simulink model "NLPIDVersion2"  (Simulink 7.3)
settings: Solver=ode5  StartTime=0.0  StopTime=inf  FixedStep=0.1  RelTol=1e-3
undefined symbols (not defined in the file): eta1_0_real, v1_0_real, velocitySatValues1
libraries: dspmtrx3 x16, simulink x14, dspindex x5, marine_gnc x4, simulink_extras x1, dspinverses x1
(part 2 of 4)

== system NLPIDVersion2/Main Subsystems/Control/Nonlinear PID/Auxiliary function g_s ==
  g_s eq : Subsystem
  g_s^q eq : Subsystem
  g_s^s eq : Subsystem
  g_s^t eq : Subsystem
  tag scope: gs=global, gs_q=global, gs_s=global, gs_t=global
  wires:
  [fs_t] -> g_s^t eq/2(f_s^t)
  g_s^t eq/1(g_a^t) -> [gs_t]
  [psiLOS_s_2] -> g_s^s eq/4(psi_los^s^2)
  [fs_s] -> g_s^s eq/3(f_s^s)
  g_s^s eq/1(g_s^s) -> [gs_s]
  g_s^q eq/1(g_s^q) -> [gs_q]
  [psiLOS_qs] -> g_s^q eq/4(psi_los^sq)
  [fs_q] -> g_s^q eq/3(f_s^q)
  g_s eq/1(g_s) -> [gs]
  [psiLOS_s] -> g_s^t eq/1(psi_los^s), g_s^s eq/2(psi_los^s), g_s^q eq/2(psi_los^s), g_s eq/2(psi_los^s)
  [fs] -> g_s^s eq/1(f_s), g_s^q eq/1(f_s), g_s eq/1(f_s)

== system NLPIDVersion2/Main Subsystems/Control/Nonlinear PID/Control law ==
  Sum : Sum  Inputs=+++  OutDataType=fixdt(1, 16)  OutScaling=2^-10
  tau_FF : Subsystem
  tau_FL : Subsystem
  tau_PID : Subsystem
  tag scope: ctrl2tau=global
  wires:
  Sum/1 -> [ctrl2tau]
  tau_PID/1(tau_PID) -> Sum/1
  tau_FL/1(tau_FL) -> Sum/2
  tau_FF/1(tau_FF) -> Sum/3

== system NLPIDVersion2/Main Subsystems/Control/Nonlinear PID/R(psi) ==
  -1 : Gain  Gain=-1  ParameterDataType=fixdt(1, 16)  ParameterScaling=2^0  OutDataType=fixdt(1, 16)  OutScaling=2^0
  Mux : Mux  Inputs=9
  R(psi) : Reshape  OutputDimensionality=Customize  OutputDimensions=[3,3]
  R11 : Trigonometry  Operator=cos
  R12 : Trigonometry
  R{13,23,31..32} (4 alike) : Constant  Value=0
  R21 : Trigonometry
  R22 : Trigonometry  Operator=cos
  R33 : Constant
  R^T : dspmtrx3/Transpose  SystemSampleTime=-1  Hermitian=off  overflowFlag=off
  psi : Selector  InputPortWidth=3  IndexOptions=Index vector (dialog)  Indices=[3]  OutputSizes=1
  tag scope: Rpsi=global, Rpsi_T=global
  wires:
  R(psi)/1 -> [Rpsi], R^T/1
  Mux/1 -> R(psi)/1
  psi/1 -> R11/1, R21/1, R12/1, R22/1
  R11/1 -> Mux/1
  R21/1 -> Mux/2
  R31/1 -> Mux/3
  R12/1 -> -1/1
  R22/1 -> Mux/5
  R32/1 -> Mux/6
  R13/1 -> Mux/7
  R33/1 -> Mux/9
  R23/1 -> Mux/8
  -1/1 -> Mux/4
  [eta] -> psi/1
  R^T/1 -> [Rpsi_T]

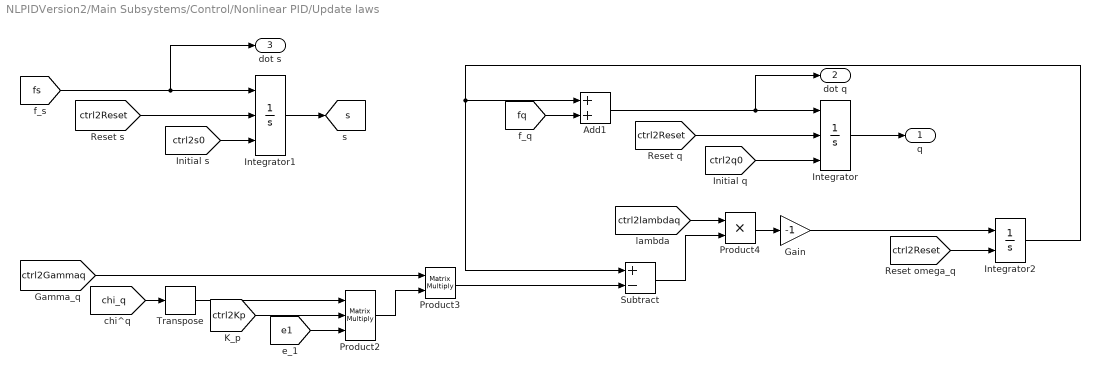
== system NLPIDVersion2/Main Subsystems/Control/Nonlinear PID/Update laws ==
  Add1 : Sum  OutDataType=fixdt(1, 16)  OutScaling=2^-10
  Gain : Gain  Gain=-1  ParameterDataType=fixdt(1, 16)  ParameterScaling=2^0  OutDataType=fixdt(1, 16)  OutScaling=2^0
  Integrator : Integrator  ExternalReset=level  InitialConditionSource=external
  Integrator1 : Integrator  ExternalReset=level  InitialConditionSource=external  InitialCondition=250
  Integrator2 : Integrator  ExternalReset=level
  Product2 : Product  Inputs=3  Multiplication=Matrix(*)  OutDataType=fixdt(1, 16)  OutScaling=2^0  RndMeth=Zero
  Product3 : Product  Multiplication=Matrix(*)  OutDataType=fixdt(1, 16)  OutScaling=2^0  RndMeth=Zero
  Product4 : Product  OutDataType=fixdt(1, 16)  OutScaling=2^0  RndMeth=Zero
  Subtract : Sum  Inputs=+-  OutDataType=fixdt(1, 16)  OutScaling=2^-10
  Transpose : dspmtrx3/Transpose  SystemSampleTime=-1  Hermitian=off  overflowFlag=off
  q : Outport  PortDimensions=2
  dot q : Outport  Port=2  PortDimensions=2
  dot s : Outport  Port=3  PortDimensions=1
  tag scope: s=global
  wires:
  [chi_q] -> Transpose/1
  [e1] -> Product2/3
  Transpose/1 -> Product2/1
  [ctrl2Kp] -> Product2/2
  [ctrl2Gammaq] -> Product3/1
  Product3/1 -> Subtract/2
  Product2/1 -> Product3/2
  [fs] -> Integrator1/1, dot s/1
  Integrator1/1 -> [s]
  [ctrl2Reset] -> Integrator1/2
  [ctrl2s0] -> Integrator1/3
  [fq] -> Add1/2
  Add1/1 -> Integrator/1, dot q/1
  [ctrl2lambdaq] -> Product4/1
  Subtract/1 -> Product4/2
  Product4/1 -> Gain/1
  Gain/1 -> Integrator2/1
  Integrator/1 -> q/1
  Integrator2/1 -> Add1/1, Subtract/1
  [ctrl2Reset] -> Integrator/2
  [ctrl2q0] -> Integrator/3
  [ctrl2Reset] -> Integrator2/2

== system NLPIDVersion2/Main Subsystems/Control/Nonlinear PID/a_d ==
  dot q : Inport
  dot s : Inport  Port=2
  Product : Product  Multiplication=Matrix(*)  OutDataType=fixdt(1, 16)  OutScaling=2^0  RndMeth=Zero
  Product1 : Product  Multiplication=Matrix(*)  OutDataType=fixdt(1, 16)  OutScaling=2^0  RndMeth=Zero
  Sum : Sum  Inputs=+++  OutDataType=fixdt(1, 16)  OutScaling=2^-10
  v_d^q : Subsystem
  v_d^s : Subsystem
  v_d^t : Subsystem
  tag scope: ad=global
  wires:
  v_d^q/1(v_d^q) -> Product/1
  dot q/1 -> Product/2
  Product/1 -> Sum/1
  v_d^s/1(v_d^s) -> Product1/1
  dot s/1 -> Product1/2
  Product1/1 -> Sum/2
  v_d^t/1(v_d^t) -> Sum/3
  Sum/1 -> [ad]
  [gq_q] -> v_d^q/1(g_q^q)
  [gs_q] -> v_d^q/2(g_s^q)
  [gq_s] -> v_d^s/1(g_q^s)
  [gs_s] -> v_d^s/2(g_s^s)
  [gq_t] -> v_d^t/1(g_q^t)
  [gs_t] -> v_d^t/2(g_s^t)

== system NLPIDVersion2/Main Subsystems/Control/Nonlinear PID/e2 ==
  Product : Product  Multiplication=Matrix(*)  OutDataType=fixdt(1, 16)  OutScaling=2^0  RndMeth=Zero
  Subtract : Sum  Inputs=+-  OutDataType=fixdt(1, 16)  OutScaling=2^-10
  tag scope: e2=global
  wires:
  [nu] -> Subtract/1
  Product/1 -> Subtract/2
  [Rpsi_T] -> Product/1
  [vd] -> Product/2
  Subtract/1 -> [e2]

== system NLPIDVersion2/Main Subsystems/Control/Nonlinear PID/e_1 ==
  Heading to -pi/pi : Subsystem
  Heading to -pi/pi1 : Subsystem
  Subtract : Sum  Inputs=+-  OutDataType=fixdt(1, 16)  OutScaling=2^-10
  tag scope: e1=global
  wires:
  Subtract/1 -> Heading to -pi/pi1/1(eta rad)
  [eta] -> Heading to -pi/pi/1(eta rad)
  Heading to -pi/pi/1(eta -pi/pi) -> Subtract/1
  Heading to -pi/pi1/1(eta -pi/pi) -> [e1]
  [chi] -> Subtract/2

== system NLPIDVersion2/Main Subsystems/Control/Nonlinear PID/v_d ==
  Add : Sum  OutDataType=fixdt(1, 16)  OutScaling=2^-10
  tag scope: vd=global
  wires:
  [gq] -> Add/1
  [gs] -> Add/2
  Add/1 -> [vd]

== system NLPIDVersion2/Main Subsystems/Control/Nonlinear PID/zeta ==
  Integrator : Integrator  ExternalReset=level  InitialCondition=[0 0 0]'
  Product : Product  Multiplication=Matrix(*)  OutDataType=fixdt(1, 16)  OutScaling=2^0  RndMeth=Zero
  tag scope: zeta=global
  wires:
  [ctrl2Reset] -> Integrator/2
  Product/1 -> Integrator/1
  Integrator/1 -> [zeta]
  [e2] -> Product/2
  [Rpsi] -> Product/1

== system NLPIDVersion2/Main Subsystems/Control/PS3 u input control/Subsystem ==
  u_act : Inport  OutDataType=fixdt(1, 16)  OutScaling=2^0
  Bus Selector : BusSelector  OutputSignals=u_1,u_2,u_3,u_4,u_5
  Mux : Mux  Inputs=5
  f_act to tau : Subsystem
  u_act to f_act : Subsystem
  tau : Outport
  wires:
  u_act/1 -> Bus Selector/1
  f_act to tau/1(tau) -> tau/1
  u_act to f_act/1(f_act) -> f_act to tau/1(f_act)
  Mux/1 -> u_act to f_act/1(u_act)
  Bus Selector/1 -> Mux/1  "<u_1>"
  Bus Selector/2 -> Mux/2  "<u_2>"
  Bus Selector/3 -> Mux/3  "<u_3>"
  Bus Selector/4 -> Mux/4  "<u_4>"
  Bus Selector/5 -> Mux/5  "<u_5>"

== system NLPIDVersion2/Main Subsystems/Control/Thruster allocation/VSP030 BT040 ==
  f_act : Inport
  BT_power_limit : Constant  Value=0.4
  Mux1 : Mux  Inputs=3
  VSP_speeds : Constant  Value=0.3
  f_act to u_act : Subsystem
  TC : Outport  OutDataType=fixdt(1, 16)  OutScaling=2^0
  wires:
  Mux1/1 -> TC/1
  f_act/1 -> f_act to u_act/1(f_act)
  BT_power_limit/1 -> Mux1/2
  VSP_speeds/1 -> Mux1/3
  f_act to u_act/1(u_act) -> Mux1/1

== system NLPIDVersion2/Main Subsystems/Control/Thruster allocation/tau to f_act ==
  tau : Inport
  Product : Product  Multiplication=Matrix(*)  OutDataType=fixdt(1, 16)  OutScaling=2^0  RndMeth=Zero
  Pseudoinverse : dspinverses/Pseudoinverse  wanterr=off
  f_act : Outport
  wires:
  [B] -> Pseudoinverse/1
  Pseudoinverse/1 -> Product/1
  tau/1 -> Product/2
  Product/1 -> f_act/1

== system NLPIDVersion2/Main Subsystems/Guidance/Line-Of-Sight Path-Following/Heading ==
  Demux : Demux  Outputs=2
  Demux1 : Demux  Outputs=2
  Demux2 : Demux  Outputs=2
  psi_d eq : Subsystem
  psi_d^s eq : Subsystem
  psi_d^s^2 eq : Subsystem
  tag scope: psid=global, psid_s=global, psid_s_2=global
  wires:
  psi_d^s eq/3(den) -> psi_d^s^2 eq/2(den)
  psi_d^s eq/2(num) -> psi_d^s^2 eq/1(num)
  Demux2/2 -> psi_d^s^2 eq/8(y_d^s^3)
  Demux2/1 -> psi_d^s^2 eq/7(x_d^s^3)
  psi_d^s^2 eq/1(psi_d^s^2) -> [psid_s_2]
  [pd_s_3] -> Demux2/1
  psi_d^s eq/1(psi_d^s) -> [psid_s]
  Demux1/2 -> psi_d^s^2 eq/6(y_d^s^2), psi_d^s eq/4(y_d^s^2)
  Demux1/1 -> psi_d^s^2 eq/5(x_d^s^2), psi_d^s eq/3(x_d^s^2)
  [pd_s_2] -> Demux1/1
  [pd_s] -> Demux/1
  Demux/2 -> psi_d^s^2 eq/4(y_d^s), psi_d^s eq/2(y_d^s), psi_d eq/2(y_d^s)
  Demux/1 -> psi_d^s^2 eq/3(x_d^s), psi_d^s eq/1(x_d^s), psi_d eq/1(x_d^s)
  psi_d eq/1(psi_d) -> [psid]

== system NLPIDVersion2/Main Subsystems/Guidance/Line-Of-Sight Path-Following/Line-Of-Sight ==
  Dynamic LOS assigment for qdot : Subsystem
  Dynamic assigment for sdot : Subsystem
  Gradient update law for sdot : Subsystem
  LOS heading : Subsystem
  Position error signals : Subsystem
  Subtract : Sum  Inputs=+-  OutDataType=fixdt(1, 16)  OutScaling=2^-10
  Virtual Vessel : Subsystem
  wires:
  Gradient update law for sdot/3(omega_s^s) -> Dynamic assigment for sdot/6(omega_s^s)
  Gradient update law for sdot/2(omega_s^q) -> Dynamic assigment for sdot/5(omega_s^q)
  Position error signals/4(epsilon_n^q) -> Dynamic assigment for sdot/1(epsilon_n^q), LOS heading/4(epsilon_n^q)
  Position error signals/3(epsilon_n^s^2) -> LOS heading/3(epsilon_n^s^2)
  Position error signals/2(epsilon_n^q^2) -> LOS heading/2(epsilon_n^q^2)
  Position error signals/1(epsilon_n^qs) -> LOS heading/1(epsilon_n^qs)
  Position error signals/5(epsilon_n^s) -> Dynamic assigment for sdot/2(epsilon_n^s), LOS heading/5(epsilon_n^s)
  Position error signals/6(epsilon_n) -> LOS heading/6(epsilon_n), Dynamic assigment for sdot/3(epsilon_n)
  Gradient update law for sdot/1(omega_s) -> Dynamic assigment for sdot/4(omega_s)
  Subtract/1 -> Position error signals/1(q - p_d), Gradient update law for sdot/1(q - p_d)
  [q] -> Subtract/1
  [pd] -> Subtract/2

== system NLPIDVersion2/Main Subsystems/Guidance/Line-Of-Sight Path-Following/Path ==
  note: Path Selector == 1: Linear path
      | Path Selector == 0: Ellipse path
  Ellipse path : Subsystem
  Path Switch workaround + limiter : Subsystem
  Straight path : Subsystem

== system NLPIDVersion2/Main Subsystems/Guidance/Line-Of-Sight Path-Following/Speed assigment ==
  Derivative : Derivative
  v_s eq : Subsystem
  v_s^s eq : Subsystem
  v_s^t eq : Subsystem
  tag scope: ud_t=global, vs=global, vs_s=global, vs_t=global
  wires:
  Derivative/1 -> v_s^t eq/2(u_d^t), [ud_t]
  v_s^t eq/1(v_s^t) -> [vs_t]
  [pd_s_2] -> v_s^s eq/4(p_d^s^2)
  [pd_s] -> v_s^s eq/3(p_d^s)
  v_s^s eq/1(v_s^s) -> [vs_s]
  [ud] -> Derivative/1, v_s^s eq/2(u_d), v_s eq/2(u_d)
  [pd_sabs] -> v_s eq/1(|p_d^s|), v_s^s eq/1(|p_d^s|), v_s^t eq/1(|p_d^s|)
  v_s eq/1(v_s) -> [vs]

== system NLPIDVersion2/Main Subsystems/Plant/CSE1 actuator/Bow Thruster ==
  Bow Thruster Direction u_5 : Inport
  Bow Thruster Power : Inport  Port=2
  Add : Sum  Inputs=+++
  BT_D_Gain1 : Gain  Gain=0.02
  BT_D_Gain2 : Gain  Gain=0.02
  BT_L_Gain1 : Gain  Gain=0.02
  BT_L_Gain2 : Gain  Gain=-0.02
  BT_Power_Offset1 : Constant  Value=0.05
  BT_Power_Offset2 : Constant  Value=0.05
  BT_Power_Offset3 : Constant  Value=0.05
  Constant : Constant  Value=0  OutDataType=fixdt(1, 16)  OutScaling=2^0
  Constant1 : Constant  Value=0  OutDataType=fixdt(1, 16)  OutScaling=2^0
  Neg : Gain  Gain=-1  ParameterDataType=fixdt(1, 16)  ParameterScaling=2^0  OutDataType=fixdt(1, 16)  OutScaling=2^0
  SIT PWM0 BT : S-Function  Priority=1  FunctionName=NI_SIT_IO  Parameters=width dtype portnum stime stype btype  EnableBusSupport=off  mask(SIT Outport){portnum=1, width=-1, stime=-1, dtype=auto, stype=auto, btype=0}
      mask prompts: portnum "Port number:"; width "Port dimensions (-1 for dynamically sized):"; stime "Sample time (-1 for inherited):"; dtype "Data type:"; stype "Signal type:"; btype "Block type:"
      mask help: Use this outport on any level of nested subsystems to allow the LabVIEW Simulation Interface Toolkit to map hardware to it.
      mask init:
      | NI_SIT_IO_init;
      settings: CopyFcn=NI_SIT_IO_callbacks(1);  DeleteFcn=NI_SIT_IO_callbacks(2);
      mask StyleString: edit,edit,edit,popup(auto|double|single|int8|uint8|int16|uint16|int32|uint32|boolean),popup(auto|real|complex),edit
      mask CallbackString: NI_SIT_IO_callbacks(3);|||NI_SIT_IO_callbacks(4);||
      mask TabNameString: Parameters,Parameters,Parameters,Parameters,Parameters,Parameters
      mask Display:
      | patch([-x x], [-y y], [.90980 .81960 .32156]);
      | plot([0 -x x 0], [rad -y y rad]);
      | fprintf('SIT%d', portnum);
  Saturation Dynamic : simulink/Discontinuities/Saturation Dynamic  SystemSampleTime=-1  OutMin=[]  OutMax=[]  OutDataTypeStr=Inherit: Same as second input  OutDataType=fixdt(1, 16)  OutScaling=2^-10  DoSatur=off
  Saturation Dynamic1 : simulink/Discontinuities/Saturation Dynamic  SystemSampleTime=-1  OutMin=[]  OutMax=[]  OutDataTypeStr=Inherit: Same as second input  OutDataType=fixdt(1, 16)  OutScaling=2^-10  DoSatur=off
  Saturation Dynamic2 : simulink/Discontinuities/Saturation Dynamic  SystemSampleTime=-1  OutMin=[]  OutMax=[]  OutDataTypeStr=Inherit: Same as second input  OutDataType=fixdt(1, 16)  OutScaling=2^-10  DoSatur=off
  Sum1 : Sum  Inputs=|++
  Sum2 : Sum  Inputs=|++
  Terminator : Terminator
  Terminator1 : Terminator
  wires:
  Bow Thruster Direction u_5/1 -> BT_D_Gain1/1, Saturation Dynamic1/2, BT_D_Gain2/1, Saturation Dynamic2/2
  BT_D_Gain1/1 -> Add/1
  BT_D_Gain2/1 -> Add/3
  BT_Power_Offset1/1 -> Add/2
  Add/1 -> Saturation Dynamic/2
  Bow Thruster Power/1 -> BT_L_Gain2/1, Saturation Dynamic2/1, BT_L_Gain1/1, Neg/1
  Sum1/1 -> Saturation Dynamic/1
  BT_L_Gain1/1 -> Sum1/1
  BT_L_Gain2/1 -> Sum2/1
  Sum2/1 -> Saturation Dynamic/3
  BT_Power_Offset2/1 -> Sum1/2
  BT_Power_Offset3/1 -> Sum2/2
  Saturation Dynamic/1 -> SIT PWM0 BT/1
  Saturation Dynamic2/1 -> Terminator1/1
  Saturation Dynamic1/1 -> Terminator/1
  Constant/1 -> Saturation Dynamic1/1
  Constant1/1 -> Saturation Dynamic2/3
  Neg/1 -> Saturation Dynamic1/3

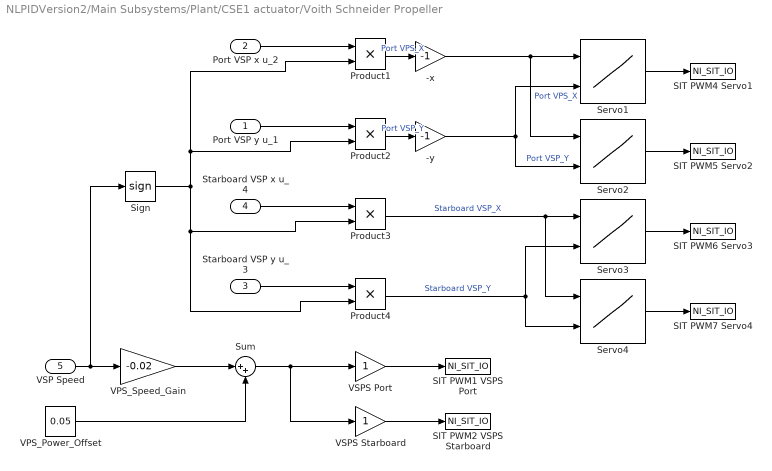
== system NLPIDVersion2/Main Subsystems/Plant/CSE1 actuator/Voith Schneider Propeller  ==
  Port VSP y u_1 : Inport
  Port VSP x u_2 : Inport  Port=2
  Starboard VSP y u_3 : Inport  Port=3
  Starboard VSP x u_4 : Inport  Port=4
  VSP Speed : Inport  Port=5
  -x : Gain  Gain=-1
  -y : Gain  Gain=-1
  Product{1..4} (4 alike) : Product  RndMeth=Zero
  SIT PWM1 VSPS Port : S-Function  Priority=5  FunctionName=NI_SIT_IO  Parameters=width dtype portnum stime stype btype  EnableBusSupport=off  mask(SIT Outport){portnum=5, width=-1, stime=-1, dtype=auto, stype=auto, btype=0}
      mask prompts: portnum "Port number:"; width "Port dimensions (-1 for dynamically sized):"; stime "Sample time (-1 for inherited):"; dtype "Data type:"; stype "Signal type:"; btype "Block type:"
      mask help: Use this outport on any level of nested subsystems to allow the LabVIEW Simulation Interface Toolkit to map hardware to it.
      mask init:
      | NI_SIT_IO_init;
      settings: CopyFcn=NI_SIT_IO_callbacks(1);  DeleteFcn=NI_SIT_IO_callbacks(2);
      mask StyleString: edit,edit,edit,popup(auto|double|single|int8|uint8|int16|uint16|int32|uint32|boolean),popup(auto|real|complex),edit
      mask CallbackString: NI_SIT_IO_callbacks(3);|||NI_SIT_IO_callbacks(4);||
      mask TabNameString: Parameters,Parameters,Parameters,Parameters,Parameters,Parameters
      mask Display:
      | patch([-x x], [-y y], [.90980 .81960 .32156]);
      | plot([0 -x x 0], [rad -y y rad]);
      | fprintf('SIT%d', portnum);
  SIT PWM2 VSPS Starboard : S-Function  Priority=6  FunctionName=NI_SIT_IO  Parameters=width dtype portnum stime stype btype  EnableBusSupport=off  mask(SIT Outport){portnum=6, width=-1, stime=-1, dtype=auto, stype=auto, btype=0}
      mask prompts: portnum "Port number:"; width "Port dimensions (-1 for dynamically sized):"; stime "Sample time (-1 for inherited):"; dtype "Data type:"; stype "Signal type:"; btype "Block type:"
      mask help: Use this outport on any level of nested subsystems to allow the LabVIEW Simulation Interface Toolkit to map hardware to it.
      mask init:
      | NI_SIT_IO_init;
      settings: CopyFcn=NI_SIT_IO_callbacks(1);  DeleteFcn=NI_SIT_IO_callbacks(2);
      mask StyleString: edit,edit,edit,popup(auto|double|single|int8|uint8|int16|uint16|int32|uint32|boolean),popup(auto|real|complex),edit
      mask CallbackString: NI_SIT_IO_callbacks(3);|||NI_SIT_IO_callbacks(4);||
      mask TabNameString: Parameters,Parameters,Parameters,Parameters,Parameters,Parameters
      mask Display:
      | patch([-x x], [-y y], [.90980 .81960 .32156]);
      | plot([0 -x x 0], [rad -y y rad]);
      | fprintf('SIT%d', portnum);
  SIT PWM4 Servo1 : S-Function  Priority=1  FunctionName=NI_SIT_IO  Parameters=width dtype portnum stime stype btype  EnableBusSupport=off  mask(SIT Outport){portnum=1, width=-1, stime=-1, dtype=auto, stype=auto, btype=0}
      mask prompts: portnum "Port number:"; width "Port dimensions (-1 for dynamically sized):"; stime "Sample time (-1 for inherited):"; dtype "Data type:"; stype "Signal type:"; btype "Block type:"
      mask help: Use this outport on any level of nested subsystems to allow the LabVIEW Simulation Interface Toolkit to map hardware to it.
      mask init:
      | NI_SIT_IO_init;
      settings: CopyFcn=NI_SIT_IO_callbacks(1);  DeleteFcn=NI_SIT_IO_callbacks(2);
      mask StyleString: edit,edit,edit,popup(auto|double|single|int8|uint8|int16|uint16|int32|uint32|boolean),popup(auto|real|complex),edit
      mask CallbackString: NI_SIT_IO_callbacks(3);|||NI_SIT_IO_callbacks(4);||
      mask TabNameString: Parameters,Parameters,Parameters,Parameters,Parameters,Parameters
      mask Display:
      | patch([-x x], [-y y], [.90980 .81960 .32156]);
      | plot([0 -x x 0], [rad -y y rad]);
      | fprintf('SIT%d', portnum);
  SIT PWM5 Servo2 : S-Function  Priority=2  FunctionName=NI_SIT_IO  Parameters=width dtype portnum stime stype btype  EnableBusSupport=off  mask(SIT Outport){portnum=2, width=-1, stime=-1, dtype=auto, stype=auto, btype=0}
      mask prompts: portnum "Port number:"; width "Port dimensions (-1 for dynamically sized):"; stime "Sample time (-1 for inherited):"; dtype "Data type:"; stype "Signal type:"; btype "Block type:"
      mask help: Use this outport on any level of nested subsystems to allow the LabVIEW Simulation Interface Toolkit to map hardware to it.
      mask init:
      | NI_SIT_IO_init;
      settings: CopyFcn=NI_SIT_IO_callbacks(1);  DeleteFcn=NI_SIT_IO_callbacks(2);
      mask StyleString: edit,edit,edit,popup(auto|double|single|int8|uint8|int16|uint16|int32|uint32|boolean),popup(auto|real|complex),edit
      mask CallbackString: NI_SIT_IO_callbacks(3);|||NI_SIT_IO_callbacks(4);||
      mask TabNameString: Parameters,Parameters,Parameters,Parameters,Parameters,Parameters
      mask Display:
      | patch([-x x], [-y y], [.90980 .81960 .32156]);
      | plot([0 -x x 0], [rad -y y rad]);
      | fprintf('SIT%d', portnum);
  SIT PWM6 Servo3 : S-Function  Priority=3  FunctionName=NI_SIT_IO  Parameters=width dtype portnum stime stype btype  EnableBusSupport=off  mask(SIT Outport){portnum=3, width=-1, stime=-1, dtype=auto, stype=auto, btype=0}
      mask prompts: portnum "Port number:"; width "Port dimensions (-1 for dynamically sized):"; stime "Sample time (-1 for inherited):"; dtype "Data type:"; stype "Signal type:"; btype "Block type:"
      mask help: Use this outport on any level of nested subsystems to allow the LabVIEW Simulation Interface Toolkit to map hardware to it.
      mask init:
      | NI_SIT_IO_init;
      settings: CopyFcn=NI_SIT_IO_callbacks(1);  DeleteFcn=NI_SIT_IO_callbacks(2);
      mask StyleString: edit,edit,edit,popup(auto|double|single|int8|uint8|int16|uint16|int32|uint32|boolean),popup(auto|real|complex),edit
      mask CallbackString: NI_SIT_IO_callbacks(3);|||NI_SIT_IO_callbacks(4);||
      mask TabNameString: Parameters,Parameters,Parameters,Parameters,Parameters,Parameters
      mask Display:
      | patch([-x x], [-y y], [.90980 .81960 .32156]);
      | plot([0 -x x 0], [rad -y y rad]);
      | fprintf('SIT%d', portnum);
  SIT PWM7 Servo4 : S-Function  Priority=4  FunctionName=NI_SIT_IO  Parameters=width dtype portnum stime stype btype  EnableBusSupport=off  mask(SIT Outport){portnum=4, width=-1, stime=-1, dtype=auto, stype=auto, btype=0}
      mask prompts: portnum "Port number:"; width "Port dimensions (-1 for dynamically sized):"; stime "Sample time (-1 for inherited):"; dtype "Data type:"; stype "Signal type:"; btype "Block type:"
      mask help: Use this outport on any level of nested subsystems to allow the LabVIEW Simulation Interface Toolkit to map hardware to it.
      mask init:
      | NI_SIT_IO_init;
      settings: CopyFcn=NI_SIT_IO_callbacks(1);  DeleteFcn=NI_SIT_IO_callbacks(2);
      mask StyleString: edit,edit,edit,popup(auto|double|single|int8|uint8|int16|uint16|int32|uint32|boolean),popup(auto|real|complex),edit
      mask CallbackString: NI_SIT_IO_callbacks(3);|||NI_SIT_IO_callbacks(4);||
      mask TabNameString: Parameters,Parameters,Parameters,Parameters,Parameters,Parameters
      mask Display:
      | patch([-x x], [-y y], [.90980 .81960 .32156]);
      | plot([0 -x x 0], [rad -y y rad]);
      | fprintf('SIT%d', portnum);
  Servo1 : Lookup2D  RowIndex=[-1,0,1]  ColumnIndex=[-1,0,1]  Table=reshape([0.06,0.0495363,0.043301,0.06,0.052446,0.043301,0.06,0.0541518,0.043301],3,3)
  Servo2 : Lookup2D  RowIndex=[-1,0,1]  ColumnIndex=[-1,0,1]  Table=reshape([0.03860880,0.0386088,0.03860880,0.0459941,0.0477243,0.0500953,0.057,0.057,0.057],3,3)
  Servo3 : Lookup2D  RowIndex=[-1,0,1]  ColumnIndex=[-1,0,1]  Table=reshape([0.0640809,0.0640809,0.0640809,0.0539629,0.0541315,0.0556492,0.0442664,0.0442664,0.0442664],3,3)
  Servo4 : Lookup2D  RowIndex=[-1,0,1]  ColumnIndex=[-1,0,1]  Table=reshape([0.0602867,0.0470489,0.0403879,0.0602867,0.049747,0.0403879,0.0602867,0.0526138,0.0403879],3,3)
  Sign : Signum
  Sum : Sum  Inputs=|++
  VPS_Power_Offset : Constant  Value=0.05
  VPS_Speed_Gain : Gain  Gain=-0.02
  VSPS Port : Gain  ParameterDataType=fixdt(1, 16)  ParameterScaling=2^0  OutDataType=fixdt(1, 16)  OutScaling=2^0
  VSPS Starboard : Gain  ParameterDataType=fixdt(1, 16)  ParameterScaling=2^0  OutDataType=fixdt(1, 16)  OutScaling=2^0
  wires:
  Sign/1 -> Product1/2, Product2/2, Product3/2, Product4/2
  Product1/1 -> -x/1  "Port VPS_X"
  Product2/1 -> -y/1  "Port VSP_Y"
  Servo1/1 -> SIT PWM4 Servo1/1
  Servo2/1 -> SIT PWM5 Servo2/1
  Product3/1 -> Servo3/1, Servo4/1  "Starboard VSP_X"
  Product4/1 -> Servo3/2, Servo4/2  "Starboard VSP_Y"
  Servo3/1 -> SIT PWM6 Servo3/1
  Servo4/1 -> SIT PWM7 Servo4/1
  VSP Speed/1 -> VPS_Speed_Gain/1, Sign/1
  VPS_Speed_Gain/1 -> Sum/1
  VPS_Power_Offset/1 -> Sum/2
  Sum/1 -> VSPS Port/1, VSPS Starboard/1
  -y/1 -> Servo2/2, Servo1/2  "Port VSP_Y"
  -x/1 -> Servo1/1, Servo2/1  "Port VPS_X"
  Starboard VSP y u_3/1 -> Product4/1
  Starboard VSP x u_4/1 -> Product3/1
  Port VSP y u_1/1 -> Product2/1
  Port VSP x u_2/1 -> Product1/1
  VSPS Port/1 -> SIT PWM1 VSPS Port/1
  VSPS Starboard/1 -> SIT PWM2 VSPS Starboard/1

== system NLPIDVersion2/Main Subsystems/Plant/Linear Simulator/Linear Vessel Dynamics ==
  note: This subsystem is a modifired version of Christoffer Throvaldsens Vessel Dynamic
  tau : Inport
  M_inv : Inport  Port=2
  D_L : Inport  Port=3
  Reset : Inport  Port=4
  eta_0 : Inport  Port=5
  nu_0 : Inport  Port=6
  Integrator : Integrator  ExternalReset=level  InitialConditionSource=external  InitialCondition=v1_0_real  UpperSaturationLimit=velocitySatValues1  LowerSaturationLimit=-1*velocitySatValues1
  Integrator1 : Integrator  ExternalReset=level  InitialConditionSource=external  InitialCondition=eta1_0_real
  Product1 : Product  Multiplication=Matrix(*)  RndMeth=Zero
  Product2 : Product  Multiplication=Matrix(*)  RndMeth=Zero
  Product3 : Product  Multiplication=Matrix(*)  RndMeth=Zero
  R(psi) : Subsystem
  Sum : Sum  Inputs=+-
  nudot : Terminator
  psi : Selector  InputPortWidth=3  IndexOptions=Index vector (dialog)  Indices=[3]  OutputSizes=1
  eta : Outport
  nu : Outport  Port=2
  etadot : Outport  Port=3
  wires:
  Sum/1 -> Product2/2
  Product2/1 -> Integrator/1, nudot/1
  Integrator/1 -> Product1/2, nu/1, Product3/2
  R(psi)/1(R) -> Product3/1
  psi/1 -> R(psi)/1(psi)
  M_inv/1 -> Product2/1
  tau/1 -> Sum/1
  Product1/1 -> Sum/2
  Product3/1 -> etadot/1, Integrator1/1
  Integrator1/1 -> psi/1, eta/1
  nu_0/1 -> Integrator/3
  Reset/1 -> Integrator/2, Integrator1/2
  eta_0/1 -> Integrator1/3
  D_L/1 -> Product1/1

== system NLPIDVersion2/Main Subsystems/Control/Nonlinear PID/Auxilary functions g_q/g_q eq ==
  f_q : Inport
  psi_los^q : Inport  Port=2
  Product : Product  Multiplication=Matrix(*)  OutDataType=fixdt(1, 16)  OutScaling=2^0  RndMeth=Zero
  Vector Concatenate : Concatenate  Mode=Vector
  g_q : Outport
  wires:
  Product/1 -> Vector Concatenate/2
  psi_los^q/1 -> Product/1
  f_q/1 -> Product/2, Vector Concatenate/1
  Vector Concatenate/1 -> g_q/1

== system NLPIDVersion2/Main Subsystems/Control/Nonlinear PID/Auxilary functions g_q/g_q^q eq ==
  f_q : Inport
  psi_los^q : Inport  Port=2
  f_q^q : Inport  Port=3
  psi_los^q^2 : Inport  Port=4
  Add : Sum  OutDataType=fixdt(1, 16)  OutScaling=2^-10
  Matrix Concatenate : Concatenate  Mode=Multidimensional array
  Product : Product  Multiplication=Matrix(*)  OutDataType=fixdt(1, 16)  OutScaling=2^0  RndMeth=Zero
  Product1 : Product  Multiplication=Matrix(*)  OutDataType=fixdt(1, 16)  OutScaling=2^0  RndMeth=Zero
  f_q^T : dspmtrx3/Transpose  SystemSampleTime=-1  Hermitian=off  overflowFlag=off
  psi_los^q^2T : dspmtrx3/Transpose  SystemSampleTime=-1  Hermitian=off  overflowFlag=off
  g_q^q : Outport
  wires:
  psi_los^q^2T/1 -> Product/2
  Product1/1 -> Add/2
  psi_los^q/1 -> Product1/1
  Product/1 -> Add/1
  psi_los^q^2/1 -> psi_los^q^2T/1
  f_q^T/1 -> Product/1
  f_q/1 -> f_q^T/1
  Add/1 -> Matrix Concatenate/2
  Matrix Concatenate/1 -> g_q^q/1
  f_q^q/1 -> Product1/2, Matrix Concatenate/1

== system NLPIDVersion2/Main Subsystems/Control/Nonlinear PID/Auxilary functions g_q/g_q^s eq ==
  f_q : Inport
  psi_los^q : Inport  Port=2
  f_q^s : Inport  Port=3
  psi_los^qs : Inport  Port=4
  Add : Sum  OutDataType=fixdt(1, 16)  OutScaling=2^-10
  Product : Product  Multiplication=Matrix(*)  OutDataType=fixdt(1, 16)  OutScaling=2^0  RndMeth=Zero
  Product1 : Product  Multiplication=Matrix(*)  OutDataType=fixdt(1, 16)  OutScaling=2^0  RndMeth=Zero
  Vector Concatenate : Concatenate  Mode=Vector
  g_q^s : Outport
  wires:
  f_q/1 -> Product/2
  psi_los^qs/1 -> Product/1
  Product1/1 -> Add/2
  psi_los^q/1 -> Product1/1
  Product/1 -> Add/1
  Add/1 -> Vector Concatenate/2
  Vector Concatenate/1 -> g_q^s/1
  f_q^s/1 -> Product1/2, Vector Concatenate/1

== system NLPIDVersion2/Main Subsystems/Control/Nonlinear PID/Auxilary functions g_q/g_q^t eq ==
  psi_los^q : Inport
  f_q^t : Inport  Port=2
  Product1 : Product  Multiplication=Matrix(*)  OutDataType=fixdt(1, 16)  OutScaling=2^0  RndMeth=Zero
  Vector Concatenate : Concatenate  Mode=Vector
  g_q^t : Outport
  wires:
  psi_los^q/1 -> Product1/1
  Product1/1 -> Vector Concatenate/2
  Vector Concatenate/1 -> g_q^t/1
  f_q^t/1 -> Product1/2, Vector Concatenate/1

== system NLPIDVersion2/Main Subsystems/Control/Nonlinear PID/Auxiliary function g_s/g_s eq ==
  f_s : Inport
  psi_los^s : Inport  Port=2
  0_2x1 : Constant  Value=[0;0]  VectorParams1D=off  OutDataType=fixdt(1, 16)  OutScaling=2^0
  Product : Product  Multiplication=Matrix(*)  OutDataType=fixdt(1, 16)  OutScaling=2^0  RndMeth=Zero
  Vector Concatenate : Concatenate  Mode=Vector
  g_s : Outport
  wires:
  0_2x1/1 -> Vector Concatenate/1
  Product/1 -> Vector Concatenate/2
  psi_los^s/1 -> Product/1
  f_s/1 -> Product/2
  Vector Concatenate/1 -> g_s/1

== system NLPIDVersion2/Main Subsystems/Control/Nonlinear PID/Auxiliary function g_s/g_s^q eq ==
  f_s : Inport
  psi_los^s : Inport  Port=2
  f_s^q : Inport  Port=3
  psi_los^sq : Inport  Port=4
  0_2x2 : Constant  Value=[0 0; 0 0]  VectorParams1D=off  OutDataType=fixdt(1, 16)  OutScaling=2^0
  Add : Sum  OutDataType=fixdt(1, 16)  OutScaling=2^-10
  Matrix Concatenate : Concatenate  Mode=Multidimensional array
  Product : Product  OutDataType=fixdt(1, 16)  OutScaling=2^0  RndMeth=Zero
  Product1 : Product  OutDataType=fixdt(1, 16)  OutScaling=2^0  RndMeth=Zero
  g_s^q : Outport
  wires:
  f_s/1 -> Product/2
  psi_los^sq/1 -> Product/1
  f_s^q/1 -> Product1/2
  0_2x2/1 -> Matrix Concatenate/1
  Product1/1 -> Add/2
  psi_los^s/1 -> Product1/1
  Product/1 -> Add/1
  Add/1 -> Matrix Concatenate/2
  Matrix Concatenate/1 -> g_s^q/1

== system NLPIDVersion2/Main Subsystems/Control/Nonlinear PID/Auxiliary function g_s/g_s^s eq ==
  f_s : Inport
  psi_los^s : Inport  Port=2
  f_s^s : Inport  Port=3
  psi_los^s^2 : Inport  Port=4
  0_2x1 : Constant  Value=[0;0]  VectorParams1D=off  OutDataType=fixdt(1, 16)  OutScaling=2^0
  Add : Sum  OutDataType=fixdt(1, 16)  OutScaling=2^-10
  Product : Product  OutDataType=fixdt(1, 16)  OutScaling=2^0  RndMeth=Zero
  Product1 : Product  OutDataType=fixdt(1, 16)  OutScaling=2^0  RndMeth=Zero
  Vector Concatenate : Concatenate  Mode=Vector
  g_s^s : Outport
  wires:
  f_s^s/1 -> Product1/2
  0_2x1/1 -> Vector Concatenate/1
  f_s/1 -> Product/2
  psi_los^s^2/1 -> Product/1
  Product1/1 -> Add/2
  psi_los^s/1 -> Product1/1
  Product/1 -> Add/1
  Add/1 -> Vector Concatenate/2
  Vector Concatenate/1 -> g_s^s/1

== system NLPIDVersion2/Main Subsystems/Control/Nonlinear PID/Auxiliary function g_s/g_s^t eq ==
  psi_los^s : Inport
  f_s^t : Inport  Port=2
  0_2x1 : Constant  Value=[0;0]  VectorParams1D=off  OutDataType=fixdt(1, 16)  OutScaling=2^0
  Product1 : Product  Multiplication=Matrix(*)  OutDataType=fixdt(1, 16)  OutScaling=2^0  RndMeth=Zero
  Vector Concatenate : Concatenate  Mode=Vector
  g_a^t : Outport
  wires:
  f_s^t/1 -> Product1/2
  0_2x1/1 -> Vector Concatenate/1
  psi_los^s/1 -> Product1/1
  Product1/1 -> Vector Concatenate/2
  Vector Concatenate/1 -> g_a^t/1

== system NLPIDVersion2/Main Subsystems/Control/Nonlinear PID/Control law/tau_FF ==
  Product : Product  Inputs=3  Multiplication=Matrix(*)  OutDataType=fixdt(1, 16)  OutScaling=2^0  RndMeth=Zero
  Product1 : Product  Inputs=4  Multiplication=Matrix(*)  OutDataType=fixdt(1, 16)  OutScaling=2^0  RndMeth=Zero
  S(r)^T : Subsystem
  Subtract : Sum  Inputs=+-  OutDataType=fixdt(1, 16)  OutScaling=2^-10
  tau_FF : Outport
  wires:
  Subtract/1 -> tau_FF/1
  [Rpsi_T] -> Product/2, Product1/3
  [ad] -> Product/3
  Product/1 -> Subtract/1
  Product1/1 -> Subtract/2
  S(r)^T/1(S(r)^T) -> Product1/2
  [vd] -> Product1/4
  [M] -> Product/1, Product1/1

== system NLPIDVersion2/Main Subsystems/Control/Nonlinear PID/Control law/tau_FL ==
  Product1 : Product  Multiplication=Matrix(*)  OutDataType=fixdt(1, 16)  OutScaling=2^0  RndMeth=Zero
  tau_FL : Outport
  wires:
  [DL] -> Product1/1
  Product1/1 -> tau_FL/1
  [nu] -> Product1/2

== system NLPIDVersion2/Main Subsystems/Control/Nonlinear PID/Control law/tau_PID ==
  Product : Product  Inputs=3  Multiplication=Matrix(*)  OutDataType=fixdt(1, 16)  OutScaling=2^0  RndMeth=Zero
  Product1 : Product  Inputs=3  Multiplication=Matrix(*)  OutDataType=fixdt(1, 16)  OutScaling=2^0  RndMeth=Zero
  Product2 : Product  Multiplication=Matrix(*)  OutDataType=fixdt(1, 16)  OutScaling=2^0  RndMeth=Zero
  Sum : Sum  Inputs=---  OutDataType=fixdt(1, 16)  OutScaling=2^-10
  tau_PID : Outport
  wires:
  [Rpsi_T] -> Product/1, Product1/1
  [ctrl2Kp] -> Product/2
  [e1] -> Product/3
  [ctrl2Ki] -> Product1/2
  [zeta] -> Product1/3
  [ctrl2Kd] -> Product2/1
  [e2] -> Product2/2
  Sum/1 -> tau_PID/1
  Product/1 -> Sum/1
  Product1/1 -> Sum/2
  Product2/1 -> Sum/3

== system NLPIDVersion2/Main Subsystems/Control/Nonlinear PID/a_d/v_d^q ==
  g_q^q : Inport
  g_s^q : Inport  Port=2
  Add : Sum  OutDataType=fixdt(1, 16)  OutScaling=2^-10
  v_d^q : Outport
  wires:
  Add/1 -> v_d^q/1
  g_q^q/1 -> Add/1
  g_s^q/1 -> Add/2

== system NLPIDVersion2/Main Subsystems/Control/Nonlinear PID/a_d/v_d^s ==
  g_q^s : Inport
  g_s^s : Inport  Port=2
  Add1 : Sum  OutDataType=fixdt(1, 16)  OutScaling=2^-10
  v_d^s : Outport
  wires:
  Add1/1 -> v_d^s/1
  g_q^s/1 -> Add1/1
  g_s^s/1 -> Add1/2

== system NLPIDVersion2/Main Subsystems/Control/Nonlinear PID/a_d/v_d^t ==
  g_q^t : Inport
  g_s^t : Inport  Port=2
  Add : Sum  OutDataType=fixdt(1, 16)  OutScaling=2^-10
  v_d^t : Outport
  wires:
  Add/1 -> v_d^t/1
  g_q^t/1 -> Add/1
  g_s^t/1 -> Add/2

== system NLPIDVersion2/Main Subsystems/Control/Nonlinear PID/e_1/Heading to -pi/pi ==
  eta rad : Inport
  Demux : Demux  Outputs=3
  Mux : Mux  Inputs=3
  rad to [-pi pi] : Subsystem
      mask Type: rad to pi/pi
      mask Description: Converts an angle in rad to between -pi and pi
      mask Display: disp('rad to [-pi pi]')
  eta -pi/pi : Outport
  wires:
  rad to [-pi pi]/1("[-pi pi]") -> Mux/3
  Mux/1 -> eta -pi/pi/1
  eta rad/1 -> Demux/1
  Demux/2 -> Mux/2
  Demux/1 -> Mux/1
  Demux/3 -> rad to [-pi pi]/1(rad)

== system NLPIDVersion2/Main Subsystems/Control/Nonlinear PID/e_1/Heading to -pi/pi1 ==
  eta rad : Inport
  Demux : Demux  Outputs=3
  Mux : Mux  Inputs=3
  rad to [-pi pi] : Subsystem
      mask Type: rad to pi/pi
      mask Description: Converts an angle in rad to between -pi and pi
      mask Display: disp('rad to [-pi pi]')
  eta -pi/pi : Outport
  wires:
  rad to [-pi pi]/1("[-pi pi]") -> Mux/3
  Mux/1 -> eta -pi/pi/1
  eta rad/1 -> Demux/1
  Demux/2 -> Mux/2
  Demux/1 -> Mux/1
  Demux/3 -> rad to [-pi pi]/1(rad)

== system NLPIDVersion2/Main Subsystems/Control/PS3 u input control/Subsystem/f_act to tau ==
  f_act : Inport
  Product : Product  Multiplication=Matrix(*)  OutDataType=fixdt(1, 16)  OutScaling=2^0  RndMeth=Zero
  T_e : Subsystem
  tau : Outport
  wires:
  f_act/1 -> Product/2
  T_e/1(T_e) -> Product/1
  Product/1 -> tau/1

== system NLPIDVersion2/Main Subsystems/Control/PS3 u input control/Subsystem/u_act to f_act ==
  u_act : Inport
  Demux : Demux  Outputs=5
  Mux : Mux  Inputs=5
  u_1 to f_1 : Lookup  InputValues=|  Table=|  LookUpMeth=Interpolation-Use End Values  OutDataType=fixdt(1, 16)  OutScaling=2^0
      InputValues=|
      | [-1.0000
      |    -0.9000
      |    -0.8000
      |    -0.7000
      |    -0.6000
      |    -0.5000
      |    -0.4000
      |    -0.3000
      |    -0.2089
      |     0.0500
      |     0.1000
      |     0.2000
      |     0.3000
      |     0.4000
      |     0.5000
      |     0.6000
      |     0.7000
      |     0.8000
      |     0.9000]
      Table=|
      | [-1.324
      | -1.169
      | -0.919
      | -0.703
      | -0.535
      | -0.292
      | -0.165
      | -0.060
      | 0.000
      | 0.000
      | 0.051
      | 0.153
      | 0.308
      | 0.480
      | 0.663
      | 0.911
      | 1.057
      | 1.221
      | 1.374]
  u_2 to f_2 : Lookup  InputValues=|  Table=|  LookUpMeth=Interpolation-Use End Values  OutDataType=fixdt(1, 16)  OutScaling=2^0
      InputValues=|
      | [-1.0000
      |    -0.9000
      |    -0.8000
      |    -0.7000
      |    -0.6000
      |    -0.5000
      |    -0.4000
      |    -0.3000
      |    -0.2000
      |    -0.1000
      |    -0.0466
      |     0.1665
      |     0.2000
      |     0.3000
      |     0.4000
      |     0.5000
      |     0.6000
      |     0.7000
      |     0.8000
      |     0.9000
      |     1.0000]
      Table=|
      | [-0.766
      | -0.649
      | -0.522
      | -0.411
      | -0.323
      | -0.246
      | -0.156
      | -0.075
      | -0.018
      | -0.006
      | 0
      | 0
      | 0.052
      | 0.207
      | 0.331
      | 0.509
      | 0.689
      | 0.829
      | 0.961
      | 1.079
      | 1.120]
  u_3 to f_3 : Lookup  InputValues=|  Table=|  LookUpMeth=Interpolation-Use End Values  OutDataType=fixdt(1, 16)  OutScaling=2^0
      InputValues=|
      | [-0.9000
      |    -0.8000
      |    -0.7000
      |    -0.6000
      |    -0.5000
      |    -0.4000
      |    -0.3000
      |    -0.2809
      |     0.0452
      |     0.1000
      |     0.2000
      |     0.3000
      |     0.4000
      |     0.5000
      |     0.6000
      |     0.7000
      |     0.8000
      |     0.9000
      |     1.0000]
      Table=|
      | [-1.291
      | -1.088
      | -0.885
      | -0.618
      | -0.403
      | -0.211
      | -0.034
      | 0.000
      | 0.000
      | 0.014
      | 0.040
      | 0.147
      | 0.302
      | 0.494
      | 0.680
      | 0.968
      | 1.111
      | 1.289
      | 1.339]
  u_4 to f_4 : Lookup  InputValues=|  Table=|  LookUpMeth=Interpolation-Use End Values  OutDataType=fixdt(1, 16)  OutScaling=2^0
      InputValues=|
      | [-0.9000
      |    -0.8000
      |    -0.7000
      |    -0.6000
      |    -0.5000
      |    -0.4000
      |    -0.3000
      |    -0.2000
      |    -0.1000
      |    -0.0674
      |     0.3588
      |     0.5000
      |     0.6000
      |     0.7000
      |     0.8000
      |     0.9000
      |     1.0000]
      Table=|
      | [-1.249
      | -1.225
      | -1.094
      | -0.896
      | -0.696
      | -0.502
      | -0.314
      | -0.169
      | -0.042
      | 0.000
      | 0.000
      | 0.063
      | 0.107
      | 0.274
      | 0.441
      | 0.599
      | 0.731]
  u_5 to f_5 : Lookup  InputValues=[-.3:0.1:.3]  Table="[-1.2630 -1.0309 -0.3808 0 0.3480  0.8290 1.0930]"  LookUpMeth=Interpolation-Use End Values  OutDataType=fixdt(1, 16)  OutScaling=2^0
  f_act : Outport
  wires:
  Demux/5 -> u_5 to f_5/1
  Demux/4 -> u_4 to f_4/1
  Demux/3 -> u_3 to f_3/1
  Demux/2 -> u_2 to f_2/1
  Demux/1 -> u_1 to f_1/1
  u_act/1 -> Demux/1
  Mux/1 -> f_act/1
  u_5 to f_5/1 -> Mux/5
  u_4 to f_4/1 -> Mux/4
  u_3 to f_3/1 -> Mux/3
  u_2 to f_2/1 -> Mux/2
  u_1 to f_1/1 -> Mux/1

== system NLPIDVersion2/Main Subsystems/Control/Thruster allocation/VSP030 BT040/f_act to u_act ==
  f_act : Inport
  Demux : Demux  Outputs=5
  Mux : Mux  Inputs=5
  f_1 to u_1 VSP speed 0.3 : Subsystem
  f_2 to u_2 VSP speed 0.3 : Subsystem
  f_3 to u_3 VSP speed 0.3 : Subsystem
  f_4 to u_4 VSP speed 0.3 : Subsystem
  f_5 to u_5 BT power 0.4 : Subsystem
  u_act : Outport
  wires:
  f_5 to u_5 BT power 0.4/1(u_5) -> Mux/5
  f_4 to u_4 VSP speed 0.3/1(u_4) -> Mux/4
  f_3 to u_3 VSP speed 0.3/1(u_3) -> Mux/3
  f_2 to u_2 VSP speed 0.3/1(u_2) -> Mux/2
  f_1 to u_1 VSP speed 0.3/1(u_1) -> Mux/1
  Demux/5 -> f_5 to u_5 BT power 0.4/1(f_5)
  Demux/4 -> f_4 to u_4 VSP speed 0.3/1(f_4)
  Demux/3 -> f_3 to u_3 VSP speed 0.3/1(f_3)
  Demux/1 -> f_1 to u_1 VSP speed 0.3/1(f_1)
  Mux/1 -> u_act/1
  f_act/1 -> Demux/1
  Demux/2 -> f_2 to u_2 VSP speed 0.3/1(f_2)

== system NLPIDVersion2/Main Subsystems/Guidance/Line-Of-Sight Path-Following/Heading/psi_d eq ==
  x_d^s : Inport
  y_d^s : Inport  Port=2
  Trigonometric Function : Trigonometry  Operator=atan2
  rad to [-pi pi] : Subsystem
      mask Type: rad to pi/pi
      mask Description: Converts an angle in rad to between -pi and pi
      mask Display: disp('[0 2pi] to [-pi pi]')
  psi_d : Outport
  wires:
  x_d^s/1 -> Trigonometric Function/2
  y_d^s/1 -> Trigonometric Function/1
  rad to [-pi pi]/1("[-pi pi]") -> psi_d/1
  Trigonometric Function/1 -> rad to [-pi pi]/1(rad)

== system NLPIDVersion2/Main Subsystems/Guidance/Line-Of-Sight Path-Following/Heading/psi_d^s eq ==
  x_d^s : Inport
  y_d^s : Inport  Port=2
  x_d^s^2 : Inport  Port=3
  y_d^s^2 : Inport  Port=4
  ( x_d^s )^2 : Math  Operator=square  OutDataType=fixdt(1, 16)  OutScaling=2^0  SaturateOnIntegerOverflow=on
  ( x_d^s )^2 + ( y_d^s )^2 : Sum  OutDataType=fixdt(1, 16)  OutScaling=2^-10
  "( x_d^s * y_d^s^2 ) - ( x_d^s^2 * y_d^s ) " : Sum  Inputs=+-  OutDataType=fixdt(1, 16)  OutScaling=2^-10
  ( y_d^s )^2 : Math  Operator=square  OutDataType=fixdt(1, 16)  OutScaling=2^0  SaturateOnIntegerOverflow=on
  Divide : Product  Inputs=*/  OutDataType=fixdt(1, 16)  OutScaling=2^-10
  x_d^s * y_d^s^2 : Product  OutDataType=fixdt(1, 16)  OutScaling=2^0  RndMeth=Zero
  x_d^s^2 * y_d^s : Product  OutDataType=fixdt(1, 16)  OutScaling=2^0  RndMeth=Zero
  psi_d^s : Outport
  num : Outport  Port=2
  den : Outport  Port=3
  wires:
  Divide/1 -> psi_d^s/1
  ( x_d^s )^2 + ( y_d^s )^2/1 -> den/1, Divide/2
  "( x_d^s * y_d^s^2 ) - ( x_d^s^2 * y_d^s ) "/1 -> num/1, Divide/1
  ( y_d^s )^2/1 -> ( x_d^s )^2 + ( y_d^s )^2/2
  ( x_d^s )^2/1 -> ( x_d^s )^2 + ( y_d^s )^2/1
  x_d^s^2 * y_d^s/1 -> "( x_d^s * y_d^s^2 ) - ( x_d^s^2 * y_d^s ) "/2
  x_d^s * y_d^s^2/1 -> "( x_d^s * y_d^s^2 ) - ( x_d^s^2 * y_d^s ) "/1
  x_d^s^2/1 -> x_d^s^2 * y_d^s/1
  y_d^s^2/1 -> x_d^s * y_d^s^2/2
  y_d^s/1 -> x_d^s^2 * y_d^s/2, ( y_d^s )^2/1
  x_d^s/1 -> x_d^s * y_d^s^2/1, ( x_d^s )^2/1

== system NLPIDVersion2/Main Subsystems/Guidance/Line-Of-Sight Path-Following/Heading/psi_d^s^2 eq ==
  num : Inport
  den : Inport  Port=2
  x_d^s : Inport  Port=3
  y_d^s : Inport  Port=4
  x_d^s^2 : Inport  Port=5
  y_d^s^2 : Inport  Port=6
  x_d^s^3 : Inport  Port=7
  y_d^s^3 : Inport  Port=8
  ( x_d^s * x_d^s^2 ) + ( x_d^s^3 * y_d^s ) : Sum  OutDataType=fixdt(1, 16)  OutScaling=2^-10
  ( x_d^s * y_d^s^3  ) - ( x_d^s^3 * y_d^s ) : Sum  Inputs=+-  OutDataType=fixdt(1, 16)  OutScaling=2^-10
  * 2 : Gain  Gain=2  ParameterDataType=fixdt(1, 16)  ParameterScaling=2^0  OutDataType=fixdt(1, 16)  OutScaling=2^0
  Divide : Product  Inputs=*/  OutDataType=fixdt(1, 16)  OutScaling=2^-10
  Product1 : Product  OutDataType=fixdt(1, 16)  OutScaling=2^0  RndMeth=Zero
  Product2 : Product  OutDataType=fixdt(1, 16)  OutScaling=2^0  RndMeth=Zero
  Subtract : Sum  Inputs=+-  OutDataType=fixdt(1, 16)  OutScaling=2^-10
  "[ ( x_d^s )^2 + ( y_d^s )^2 ]^2" : Math  Operator=square  OutDataType=fixdt(1, 16)  OutScaling=2^0  SaturateOnIntegerOverflow=on
  x_d^s * x_d^s^2 : Product  OutDataType=fixdt(1, 16)  OutScaling=2^0  RndMeth=Zero
  "x_d^s * y_d^s^3 " : Product  OutDataType=fixdt(1, 16)  OutScaling=2^0  RndMeth=Zero
  x_d^s^3 * y_d^s : Product  OutDataType=fixdt(1, 16)  OutScaling=2^0  RndMeth=Zero
  y_d^s * y_d^s^2 : Product  OutDataType=fixdt(1, 16)  OutScaling=2^0  RndMeth=Zero
  psi_d^s^2 : Outport
  wires:
  Divide/1 -> psi_d^s^2/1
  "[ ( x_d^s )^2 + ( y_d^s )^2 ]^2"/1 -> Divide/2
  Subtract/1 -> Divide/1
  Product2/1 -> Subtract/2
  * 2/1 -> Product2/2
  ( x_d^s * x_d^s^2 ) + ( x_d^s^3 * y_d^s )/1 -> * 2/1
  num/1 -> Product2/1
  y_d^s^2/1 -> y_d^s * y_d^s^2/2
  y_d^s * y_d^s^2/1 -> ( x_d^s * x_d^s^2 ) + ( x_d^s^3 * y_d^s )/2
  x_d^s * x_d^s^2/1 -> ( x_d^s * x_d^s^2 ) + ( x_d^s^3 * y_d^s )/1
  x_d^s^2/1 -> x_d^s * x_d^s^2/2
  Product1/1 -> Subtract/1
  den/1 -> "[ ( x_d^s )^2 + ( y_d^s )^2 ]^2"/1, Product1/2
  ( x_d^s * y_d^s^3  ) - ( x_d^s^3 * y_d^s )/1 -> Product1/1
  x_d^s^3 * y_d^s/1 -> ( x_d^s * y_d^s^3  ) - ( x_d^s^3 * y_d^s )/2
  "x_d^s * y_d^s^3 "/1 -> ( x_d^s * y_d^s^3  ) - ( x_d^s^3 * y_d^s )/1
  y_d^s/1 -> y_d^s * y_d^s^2/1, x_d^s^3 * y_d^s/2
  x_d^s^3/1 -> x_d^s^3 * y_d^s/1
  y_d^s^3/1 -> "x_d^s * y_d^s^3 "/2
  x_d^s/1 -> x_d^s * x_d^s^2/1, "x_d^s * y_d^s^3 "/1

== system NLPIDVersion2/Main Subsystems/Guidance/Line-Of-Sight Path-Following/Line-Of-Sight/Dynamic LOS assigment for qdot ==
  f_q eq : Subsystem
  f_q^q eq : Subsystem
  f_q^s eq : Subsystem
  f_q^t eq : Subsystem
  tag scope: fq=global, fq_q=global, fq_s=global, fq_t=global
  wires:
  [ud_t] -> f_q^t eq/2(u_d^t)
  f_q^t eq/1(f_q^t) -> [fq_t]
  [psiLOS_s] -> f_q^s eq/3(psi_los^s)
  f_q^s eq/1(f_q^s) -> [fq_s]
  f_q^q eq/1("f_q^q ") -> [fq_q]
  [psiLOS_q] -> f_q^q eq/3(psi_los^q)
  f_q eq/1(f_q) -> [fq]
  [ud] -> f_q^s eq/2(u_d), f_q^q eq/2(u_d), f_q eq/2(u_d)
  [psiLOS] -> f_q^t eq/1(psi_los), f_q^s eq/1(psi_los), f_q^q eq/1(psi_los), f_q eq/1(psi_los)

== system NLPIDVersion2/Main Subsystems/Guidance/Line-Of-Sight Path-Following/Line-Of-Sight/Dynamic assigment for sdot ==
  epsilon_n^q : Inport
  epsilon_n^s : Inport  Port=2
  epsilon_n : Inport  Port=3
  omega_s : Inport  Port=4
  omega_s^q : Inport  Port=5
  omega_s^s : Inport  Port=6
  f_s eq : Subsystem
  f_s^q eq : Subsystem
  f_s^s eq : Subsystem
  f_s^t eq : Subsystem
  tag scope: fs=global, fs_q=global, fs_s=global, fs_t=global
  wires:
  [vs_t] -> f_s^t eq/3(v_s^t)
  [vs_s] -> f_s^s eq/6(v_s^s)
  epsilon_n^s/1 -> f_s^s eq/5(epsilon_n^s)
  omega_s^s/1 -> f_s^s eq/4(omega_s^s)
  epsilon_n^q/1 -> f_s^q eq/5(epsilon_n^q)
  omega_s^q/1 -> f_s^q eq/4(omega_s^q)
  omega_s/1 -> f_s eq/4(omega_s)
  [vs] -> f_s^s eq/3(v_s), f_s^q eq/3(v_s), f_s eq/3(v_s)
  epsilon_n/1 -> f_s^t eq/2(epsilon_n), f_s^s eq/2(epsilon_n), f_s^q eq/2(epsilon_n), f_s eq/2(epsilon_n)
  [Delta] -> f_s^t eq/1(Delta), f_s^s eq/1(Delta), f_s^q eq/1(Delta), f_s eq/1(Delta)
  f_s eq/1(f_s) -> [fs]
  f_s^q eq/1(f_s^q) -> [fs_q]
  f_s^s eq/1(f_s^s) -> [fs_s]
  f_s^t eq/1(f_s^t) -> [fs_t]

== system NLPIDVersion2/Main Subsystems/Guidance/Line-Of-Sight Path-Following/Line-Of-Sight/Gradient update law for sdot ==
  q - p_d : Inport  OutDataType=fixdt(1, 16)  OutScaling=2^0
  omega_s eq : Subsystem
  omega_s^q eq : Subsystem
  omega_s^s eq : Subsystem
  omega_s : Outport
  omega_s^q : Outport  Port=2
  omega_s^s : Outport  Port=3
  wires:
  q - p_d/1 -> omega_s^s eq/2(q - p_d), omega_s eq/2(q - p_d)
  omega_s^s eq/1(omega_s^s) -> omega_s^s/1
  omega_s^q eq/1(omega_s^q) -> omega_s^q/1
  omega_s eq/1(omega_s) -> omega_s/1
  [pd_sabs] -> omega_s eq/4(|p_d^s|), omega_s^s eq/4(|p_d^s|), omega_s^q eq/3(|p_d^s|)
  [my] -> omega_s eq/3(my), omega_s^s eq/3(my), omega_s^q eq/2(my)
  [pd_s] -> omega_s^s eq/1(p_d^s), omega_s^q eq/1(p_d^s), omega_s eq/1(p_d^s)
  [pd_s_2] -> omega_s^s eq/5(p_d^s^2)

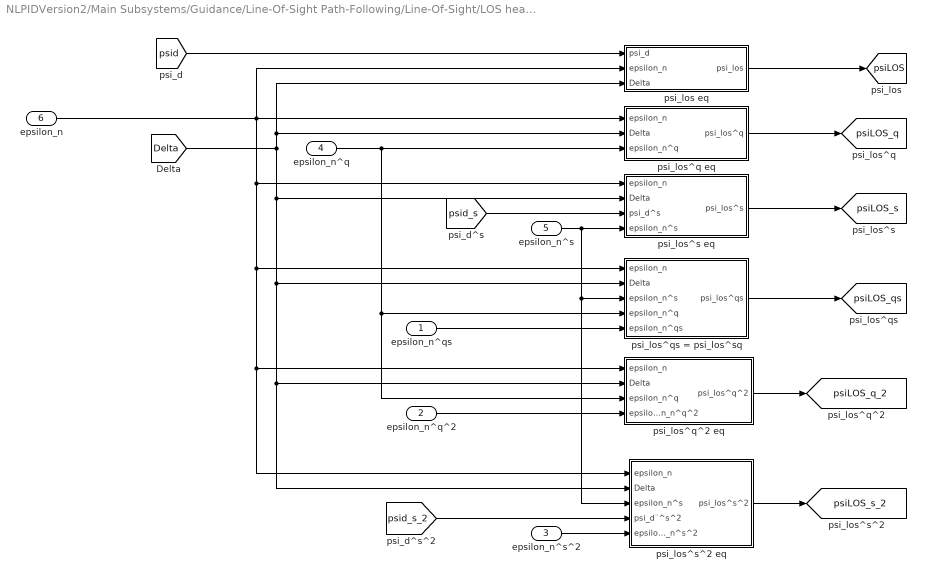
== system NLPIDVersion2/Main Subsystems/Guidance/Line-Of-Sight Path-Following/Line-Of-Sight/LOS heading ==
  epsilon_n^qs : Inport
  epsilon_n^q^2 : Inport  Port=2
  epsilon_n^s^2 : Inport  Port=3
  epsilon_n^q : Inport  Port=4
  epsilon_n^s : Inport  Port=5
  epsilon_n : Inport  Port=6
  psi_los eq : Subsystem
  psi_los^q eq : Subsystem
  psi_los^q^2 eq : Subsystem
  psi_los^qs = psi_los^sq : Subsystem
  psi_los^s eq : Subsystem
  psi_los^s^2 eq : Subsystem
  tag scope: psiLOS=global, psiLOS_q=global, psiLOS_q_2=global, psiLOS_qs=global, psiLOS_s=global, psiLOS_s_2=global
  wires:
  psi_los^s^2 eq/1(psi_los^s^2) -> [psiLOS_s_2]
  epsilon_n^s^2/1 -> psi_los^s^2 eq/5(epsilon_n^s^2)
  [psid_s_2] -> psi_los^s^2 eq/4(psi_d¨^s^2)
  epsilon_n^q^2/1 -> psi_los^q^2 eq/4(epsilon_n^q^2)
  psi_los^q^2 eq/1(psi_los^q^2) -> [psiLOS_q_2]
  epsilon_n^qs/1 -> psi_los^qs = psi_los^sq/5(epsilon_n^qs)
  epsilon_n^s/1 -> psi_los^s eq/4(epsilon_n^s), psi_los^s^2 eq/3(epsilon_n^s), psi_los^qs = psi_los^sq/3(epsilon_n^s)
  psi_los^qs = psi_los^sq/1(psi_los^qs) -> [psiLOS_qs]
  [psid_s] -> psi_los^s eq/3(psi_d^s)
  psi_los^s eq/1(psi_los^s) -> [psiLOS_s]
  psi_los^q eq/1(psi_los^q) -> [psiLOS_q]
  epsilon_n^q/1 -> psi_los^q eq/3(epsilon_n^q), psi_los^q^2 eq/3(epsilon_n^q), psi_los^qs = psi_los^sq/4(epsilon_n^q)
  [Delta] -> psi_los^q eq/2(Delta), psi_los^s eq/2(Delta), psi_los^qs = psi_los^sq/2(Delta), psi_los^s^2 eq/2(Delta), psi_los^q^2 eq/2(Delta), psi_los eq/3(Delta)
  epsilon_n/1 -> psi_los^q eq/1(epsilon_n), psi_los^s eq/1(epsilon_n), psi_los^qs = psi_los^sq/1(epsilon_n), psi_los^s^2 eq/1(epsilon_n), psi_los^q^2 eq/1(epsilon_n), psi_los eq/2(epsilon_n)
  [psid] -> psi_los eq/1(psi_d)
  psi_los eq/1(psi_los) -> [psiLOS]

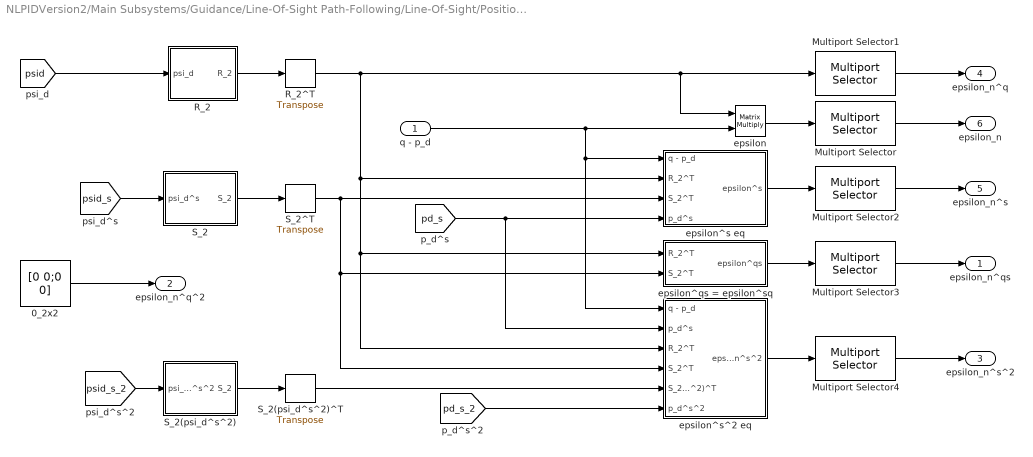
== system NLPIDVersion2/Main Subsystems/Guidance/Line-Of-Sight Path-Following/Line-Of-Sight/Position error signals ==
  q - p_d : Inport  OutDataType=fixdt(1, 16)  OutScaling=2^0
  0_2x2 : Constant  Value=[0 0;0 0]  OutDataType=fixdt(1, 16)  OutScaling=2^0
  Multiport Selector{,1..4} (5 alike) : dspindex/Multiport Selector  rowsOrCols=Rows  idxCellArray={2}  idxErrMode=Clip Index
  R_2 : Subsystem  TreatAsAtomicUnit=on
      settings: MinAlgLoopOccurrences=on
  R_2^T : dspmtrx3/Transpose  SystemSampleTime=-1  Hermitian=off  overflowFlag=off
  S_2 : Subsystem  TreatAsAtomicUnit=on
      settings: MinAlgLoopOccurrences=on
  S_2(psi_d^s^2) : Subsystem  TreatAsAtomicUnit=on
      settings: MinAlgLoopOccurrences=on
  S_2(psi_d^s^2)^T : dspmtrx3/Transpose  SystemSampleTime=-1  Hermitian=off  overflowFlag=off
  S_2^T : dspmtrx3/Transpose  SystemSampleTime=-1  Hermitian=off  overflowFlag=off
  epsilon : Product  Multiplication=Matrix(*)  OutDataType=fixdt(1, 16)  OutScaling=2^0  RndMeth=Zero
  epsilon^qs = epsilon^sq : Subsystem
  epsilon^s eq : Subsystem
  epsilon^s^2 eq : Subsystem
  epsilon_n^qs : Outport
  epsilon_n^q^2 : Outport  Port=2
  epsilon_n^s^2 : Outport  Port=3
  epsilon_n^q : Outport  Port=4
  epsilon_n^s : Outport  Port=5
  epsilon_n : Outport  Port=6
  wires:
  Multiport Selector1/1 -> epsilon_n^q/1
  [pd_s_2] -> epsilon^s^2 eq/6(p_d^s^2)
  S_2(psi_d^s^2)^T/1 -> epsilon^s^2 eq/5(S_2(psi_d^s^2)^T)
  Multiport Selector4/1 -> epsilon_n^s^2/1
  epsilon^s^2 eq/1(epsilon^s^2) -> Multiport Selector4/1
  S_2(psi_d^s^2)/1(S_2) -> S_2(psi_d^s^2)^T/1
  Multiport Selector3/1 -> epsilon_n^qs/1
  Multiport Selector2/1 -> epsilon_n^s/1
  Multiport Selector/1 -> epsilon_n/1
  epsilon/1 -> Multiport Selector/1
  0_2x2/1 -> epsilon_n^q^2/1
  epsilon^qs = epsilon^sq/1(epsilon^qs) -> Multiport Selector3/1
  S_2^T/1 -> epsilon^s^2 eq/4(S_2^T), epsilon^qs = epsilon^sq/2(S_2^T), epsilon^s eq/3(S_2^T)
  epsilon^s eq/1(epsilon^s) -> Multiport Selector2/1
  [pd_s] -> epsilon^s^2 eq/2(p_d^s), epsilon^s eq/4(p_d^s)
  S_2/1(S_2) -> S_2^T/1
  q - p_d/1 -> epsilon^s^2 eq/1(q - p_d), epsilon^s eq/1(q - p_d), epsilon/2
  R_2^T/1 -> epsilon^s^2 eq/3(R_2^T), epsilon^qs = epsilon^sq/1(R_2^T), epsilon^s eq/2(R_2^T), Multiport Selector1/1, epsilon/1
  [psid] -> R_2/1(psi_d)
  R_2/1(R_2) -> R_2^T/1
  [psid_s] -> S_2/1(psi_d^s)
  [psid_s_2] -> S_2(psi_d^s^2)/1(psi_d^s^2)
